simulink model "BMS_M0_pack_day4"  (R2026a)
settings: Solver=VariableStepAuto  AbsTol=1e-3  EnableMultiTasking=on
undefined symbols (not defined in the file or in its folder): bat, mcu
libraries: fl_lib x22, nesl_utility x18, batteryecm_lib x6, ee_lib x4, simulink x1
(part 2 of 2)

== matlab function BMS_M0_pack_day4/MATLAB Function ==
  data: cmd_preA output; tapsA input; cmd_mainA output; cmd_preB output; tapsB input; socA input; socB input; cmd_mainB output; cmd_load output; state_out output; fault_out output; Vbus input; iA input; iB input; dbg output; tempA input; tempB input
function [cmd_preA, cmd_mainA, cmd_preB, cmd_mainB, cmd_load, ...
          state_out, fault_out, dbg] = ...
         bms_reconfig_pass4(tapsA, tapsB, socA, socB, Vbus, iA, iB, ...
                            tempA, tempB)
%BMS_RECONFIG_PASS4  SOC/SOA-driven string-level reconfiguration controller.
%
%  ====================================================================
%  PROPRIETARY -- this file contains the novel contribution of this
%  project: dynamic string connect/disconnect/precharge for fault
%  isolation and SOC-driven wear levelling in a reconfigurable 3S2P pack.
%  Do not paste this logic into generic BMS code templates.
%  ====================================================================
%
%  MILESTONE 0 -- PASS 4 (final for M0).
%
%  REVISION HISTORY
%    Rev 1  SOA + topology logic.
%    Rev 2  Weld detection gated on precharge (Rev 1 tripped F_WELD_A on
%           startup because precharge current flows while the main pair is
%           deliberately open). SOC rejoin hysteresis actually applied --
%           Rev 1 rejoined at gap <= SPLIT_TH instead of < REJOIN_TH, so
%           the hysteresis band did nothing.
%    Rev 3  Warm-parallel guard reformulated. The 0.1 V rule is retained
%           for cold start, but under load the terminal difference between
%           strings is dominated by IR drop rather than stored-energy
%           mismatch, so it can never be satisfied. Bounded inrush is the
%           physically meaningful criterion. MEASURED Scenario 3: join at
%           dV = 0.149 V, inrush 1.5 A -> I_JOIN_MAX = 6 A gives 4x margin
%           while still blocking the 6.9 A cold-parallel case.
%    Rev 4  Overtemperature added (this file).
%
%  DESIGN RULES (from project brief, enforced in this order):
%    1. SOA checks run BEFORE any efficiency or balancing logic.
%    2. Break-before-make on every topology change.
%    3. Never parallel two strings unless the resulting inrush is bounded
%       (see Rev 3 note -- the original 0.1 V form is kept for cold start).
%    4. Minimum cooldown between topology changes (anti-oscillation).
%    5. Power-up / reset default is ALL SWITCHES OPEN.
%    6. Every switching action is validated by reading back current.
%
%  INPUTS
%    tapsA, tapsB  3x1  quantised tap voltages, referenced to pack negative
%    socA, socB    1x1  COULOMB-COUNTED estimates. Never true SOC.
%    Vbus          1x1  bus voltage (measured)
%    iA, iB        1x1  per-string current (measured, + = discharge)
%    tempA, tempB  3x1  per-cell temperature (deg C).
%                       INJECTED forcing function, not a thermal model --
%                       see M0 Day 1 scope decision. M0 makes NO claim
%                       about temperature reduction; that is bench-measured
%                       in M4.
%
%  OUTPUTS
%    cmd_preA/B    0/1  precharge bypass switch per string
%    cmd_mainA/B   0/1  main back-to-back pair per string
%    cmd_load      0/1  load disconnect switch
%    state_out          state code
%    fault_out          latched fault bitfield
%    dbg          10x1  diagnostics

%% ---- CONSTANTS ------------------------------------------------------
% KEEP IN SYNC WITH BMS_params.m -- a MATLAB Function block cannot read
% the base workspace.
DT              = 0.100;  % s   control loop period
V_UV_TRIP       = 2.50;   % V   [VERIFIED] SPEC pack design guideline, NCA
V_OV_TRIP       = 4.20;   % V   [VERIFIED] SPEC 3.3
I_OC_TRIP       = 12.0;   % A   [ASSUMPTION] per string, below the 15 A
                          %     cell rating with margin
T_OT_TRIP       = 60.0;   % C   [DESIGN] SPEC recommends re-discharge
                          %     release below 60 C. INTRO p.6 shows a 10 A
                          %     discharge reaching 60.9 C -- i.e. exactly
                          %     the single-string fault-mode operating
                          %     point, so this threshold is meaningful
                          %     rather than arbitrary.
T_OT_WARN       = 50.0;   % C   [ASSUMPTION] early-warning margin
DV_PARALLEL_MAX = 0.10;   % V   [ASSUMPTION] cold-start parallel limit
I_JOIN_MAX      = 6.0;    % A   [MEASURED-derived] Scenario 3 joined at
                          %     1.5 A; 6 A is 4x that and still blocks the
                          %     6.9 A unbalanced-warm-join case
R_STRING        = 0.100;  % ohm [CALCULATED] 3*20 mOhm cells + 2*20 mOhm
                          %     back-to-back MOSFET pair
T_COOLDOWN      = 0.50;   % s   [ASSUMPTION] min between topology changes
T_PRECHARGE_MAX = 0.50;   % s   [CALCULATED] 5*tau = 50 ms at R_pre = 10
                          %     ohm, C_bus = 1000 uF; 10x margin
VBUS_PRE_FRAC   = 0.95;   % fraction of string voltage = precharge done
SOC_SPLIT_TH    = 0.15;   % [DESIGN] gap at which we stop paralleling
SOC_REJOIN_TH   = 0.05;   % [DESIGN] hysteresis band for rejoining
DEBOUNCE_N      = 3;      % consecutive samples before a fault latches
VALIDATE_N      = 5;      % samples allowed for a switch to prove it moved
I_CONDUCT_MIN   = 0.20;   % A   above this counts as "current flowing"
STARTUP_N       = 10;     % ignore SOA for first 1 s while Simscape settles

%% ---- STATE CODES ----------------------------------------------------
S_INIT     = 0;   S_PRE_A    = 1;   S_PRE_B    = 2;
S_SINGLE_A = 3;   S_SINGLE_B = 4;   S_BOTH     = 5;
S_SHUTDOWN = 6;

%% ---- FAULT BITS -----------------------------------------------------
F_NONE   = 0;
F_UV_A   = 1;     F_UV_B   = 2;
F_OV_A   = 4;     F_OV_B   = 8;
F_OC_A   = 16;    F_OC_B   = 32;
F_PRE_A  = 64;    F_PRE_B  = 128;
F_WELD_A = 256;   F_WELD_B = 512;
F_OPEN_A = 1024;  F_OPEN_B = 2048;
F_OT_A   = 4096;  F_OT_B   = 8192;    % overtemperature

%% ---- PERSISTENT STATE ----------------------------------------------
persistent state fault
persistent uvA_c uvB_c ovA_c ovB_c ocA_c ocB_c otA_c otB_c
persistent t_state t_cool startup_c
persistent last_mainA last_mainB last_preA last_preB validate_c

if isempty(state)
    % POWER-UP DEFAULT: everything open. Mirrors the 100k base pull-downs
    % on the 2N2222A drivers -- on reset or brownout the hardware holds
    % the MOSFETs off, and the controller agrees.
    state = S_INIT;  fault = F_NONE;
    uvA_c = 0; uvB_c = 0; ovA_c = 0; ovB_c = 0;
    ocA_c = 0; ocB_c = 0; otA_c = 0; otB_c = 0;
    t_state = 0; t_cool = 0; startup_c = 0;
    last_mainA = 0; last_mainB = 0;
    last_preA  = 0; last_preB  = 0;
    validate_c = 0;
end

startup_c = startup_c + 1;
t_state   = t_state + DT;
if t_cool > 0, t_cool = t_cool - DT; end

%% ---- RECONSTRUCT PER-CELL VOLTAGES ---------------------------------
% The firmware performs this same subtraction: the dividers measure taps
% relative to pack negative, not individual cells. Measured reconstruction
% error 0.39 mV typical, ~7 mV worst case (2 LSB at 3.46 mV/LSB).
vA = [ tapsA(1); tapsA(2)-tapsA(1); tapsA(3)-tapsA(2) ];
vB = [ tapsB(1); tapsB(2)-tapsB(1); tapsB(3)-tapsB(2) ];

vStringA = tapsA(3);
vStringB = tapsB(3);

tMaxA = max(tempA);
tMaxB = max(tempB);

%% ---- STARTUP GRACE --------------------------------------------------
if startup_c < STARTUP_N
    cmd_preA = 0; cmd_mainA = 0;
    cmd_preB = 0; cmd_mainB = 0; cmd_load = 0;
    state_out = S_INIT; fault_out = F_NONE;
    dbg = [vA(1); vA(2); vA(3); vB(1); vB(2); vB(3); 0; 0; tMaxA; tMaxB];
    return
end

%% =====================================================================
%  LAYER 1 -- SOA CHECKS. These run first, always, and override
%  everything below.
%  =====================================================================
if any(vA < V_UV_TRIP),  uvA_c = uvA_c + 1; else, uvA_c = 0; end
if any(vB < V_UV_TRIP),  uvB_c = uvB_c + 1; else, uvB_c = 0; end
if any(vA > V_OV_TRIP),  ovA_c = ovA_c + 1; else, ovA_c = 0; end
if any(vB > V_OV_TRIP),  ovB_c = ovB_c + 1; else, ovB_c = 0; end
if abs(iA) > I_OC_TRIP,  ocA_c = ocA_c + 1; else, ocA_c = 0; end
if abs(iB) > I_OC_TRIP,  ocB_c = ocB_c + 1; else, ocB_c = 0; end
if tMaxA   > T_OT_TRIP,  otA_c = otA_c + 1; else, otA_c = 0; end
if tMaxB   > T_OT_TRIP,  otB_c = otB_c + 1; else, otB_c = 0; end

% Faults LATCH. An unloaded cell recovers voltage and would look healthy
% again; a cell removed from a heat source cools. Re-closing on either
% would oscillate the pack.
if uvA_c >= DEBOUNCE_N, fault = bitor(fault, F_UV_A); end
if uvB_c >= DEBOUNCE_N, fault = bitor(fault, F_UV_B); end
if ovA_c >= DEBOUNCE_N, fault = bitor(fault, F_OV_A); end
if ovB_c >= DEBOUNCE_N, fault = bitor(fault, F_OV_B); end
if ocA_c >= DEBOUNCE_N, fault = bitor(fault, F_OC_A); end
if ocB_c >= DEBOUNCE_N, fault = bitor(fault, F_OC_B); end
if otA_c >= DEBOUNCE_N, fault = bitor(fault, F_OT_A); end
if otB_c >= DEBOUNCE_N, fault = bitor(fault, F_OT_B); end

%% ---- STATE VALIDATION ----------------------------------------------
% A MOSFET welded closed is invisible to voltage sensing -- only current
% reveals it. Gate on the PREVIOUS cycle's precharge command: while a
% precharge switch is closed the main pair is deliberately open yet
% current legitimately flows through R_pre, which is otherwise
% indistinguishable from a weld.
in_precharge = (last_preA == 1) || (last_preB == 1);

if ~in_precharge && last_mainA == 0 && abs(iA) > I_CONDUCT_MIN
    fault = bitor(fault, F_WELD_A);
end
if ~in_precharge && last_mainB == 0 && abs(iB) > I_CONDUCT_MIN
    fault = bitor(fault, F_WELD_B);
end

% Commanded closed but no current -- only meaningful once the load is on
% and the state has settled.
if (state == S_BOTH || state == S_SINGLE_A) && last_mainA == 1 && ...
        abs(iA) < I_CONDUCT_MIN && t_state > 1.0
    validate_c = validate_c + 1;
    if validate_c >= VALIDATE_N, fault = bitor(fault, F_OPEN_A); end
elseif (state == S_BOTH || state == S_SINGLE_B) && last_mainB == 1 && ...
        abs(iB) < I_CONDUCT_MIN && t_state > 1.0
    validate_c = validate_c + 1;
    if validate_c >= VALIDATE_N, fault = bitor(fault, F_OPEN_B); end
else
    validate_c = 0;
end

faultA = bitand(fault, F_UV_A + F_OV_A + F_OC_A + F_OT_A + ...
                       F_PRE_A + F_WELD_A + F_OPEN_A) ~= 0;
faultB = bitand(fault, F_UV_B + F_OV_B + F_OC_B + F_OT_B + ...
                       F_PRE_B + F_WELD_B + F_OPEN_B) ~= 0;

%% =====================================================================
%  LAYER 2 -- BALANCING PREFERENCE (secondary; never overrides Layer 1)
%
%  A 2S string cannot be paralleled with a 3S string, so per-cell bypass
%  is unavailable. String-level selection is the only lever: run the
%  fuller string alone and let the emptier one rest.
%
%  MEASURED BEHAVIOUR (Scenario 3): from a 15% gap, single-string
%  operation closed the gap to 5% in 224 s, at which point the strings
%  rejoined. After rejoining the gap continued to zero WITHOUT controller
%  action -- paralleled strings self-balance through the bus. The value of
%  the split is therefore SAFE CONNECTION of mismatched strings, not extra
%  extracted energy. Do not claim the latter.
%  =====================================================================
soc_gap = socA - socB;
prefer_A_only = (soc_gap >  SOC_SPLIT_TH);
prefer_B_only = (soc_gap < -SOC_SPLIT_TH);
rejoin_ok     = (abs(soc_gap) < SOC_REJOIN_TH);

%% =====================================================================
%  LAYER 3 -- TRANSITION GUARDS
%  =====================================================================
% Cold start (load off, bus near 0 V): terminal dV is the right check.
% Warm parallel (load on): terminal dV is dominated by IR drop from the
% loaded string, not by stored-energy mismatch, so it can never fall below
% 0.1 V. Bound the resulting inrush instead -- that is the quantity the
% original rule was a proxy for.
dV_terminal = abs(vStringA - vStringB);
inrush_est  = dV_terminal / R_STRING;
dV_ok       = (dV_terminal < DV_PARALLEL_MAX) || (inrush_est < I_JOIN_MAX);

cool_ok   = (t_cool <= 0);
new_state = state;

switch state

    case S_INIT
        if     faultA && faultB, new_state = S_SHUTDOWN;
        elseif ~faultA,          new_state = S_PRE_A;
        elseif ~faultB,          new_state = S_PRE_B;
        else,                    new_state = S_SHUTDOWN;
        end

    case S_PRE_A
        % Bus charges through R_pre with the load disconnected. Only once
        % it has risen does the main pair close -- this is what keeps the
        % handover near 1 A instead of the measured 219 A cold-connect.
        if faultA
            new_state = S_SHUTDOWN;
        elseif Vbus >= VBUS_PRE_FRAC * vStringA
            new_state = S_SINGLE_A;
        elseif t_state > T_PRECHARGE_MAX
            fault = bitor(fault, F_PRE_A);
            new_state = S_SHUTDOWN;
        end

    case S_PRE_B
        if faultB
            new_state = S_SINGLE_A;
        elseif Vbus >= VBUS_PRE_FRAC * vStringB
            new_state = S_BOTH;
        elseif t_state > T_PRECHARGE_MAX
            fault = bitor(fault, F_PRE_B);
            new_state = S_SINGLE_A;
        end

    case S_SINGLE_A
        if     faultA && faultB,      new_state = S_SHUTDOWN;
        elseif faultA,                new_state = S_PRE_B;
        elseif ~faultB && cool_ok && dV_ok && rejoin_ok
                                      new_state = S_PRE_B;
        end

    case S_SINGLE_B
        if     faultA && faultB,      new_state = S_SHUTDOWN;
        elseif faultB,                new_state = S_PRE_A;
        elseif ~faultA && cool_ok && dV_ok && rejoin_ok
                                      new_state = S_PRE_A;
        end

    case S_BOTH
        if     faultA && faultB,         new_state = S_SHUTDOWN;
        elseif faultA,                   new_state = S_SINGLE_B;
        elseif faultB,                   new_state = S_SINGLE_A;
        elseif cool_ok && prefer_A_only, new_state = S_SINGLE_A;
        elseif cool_ok && prefer_B_only, new_state = S_SINGLE_B;
        end

    case S_SHUTDOWN
        % TERMINAL. Auto-recovery from an unknown fault is not defensible.

    otherwise
        new_state = S_SHUTDOWN;
end

if new_state ~= state
    state   = new_state;
    t_state = 0;
    t_cool  = T_COOLDOWN;
end

%% ---- OUTPUTS -------------------------------------------------------
% BREAK-BEFORE-MAKE is structural: no state asserts a precharge switch and
% its own main pair simultaneously.
switch state
    case S_INIT
        cmd_preA=0; cmd_mainA=0; cmd_preB=0; cmd_mainB=0; cmd_load=0;
    case S_PRE_A
        cmd_preA=1; cmd_mainA=0; cmd_preB=0; cmd_mainB=0; cmd_load=0;
    case S_SINGLE_A
        cmd_preA=0; cmd_mainA=1; cmd_preB=0; cmd_mainB=0; cmd_load=1;
    case S_PRE_B
        cmd_preA=0; cmd_mainA=1; cmd_preB=1; cmd_mainB=0; cmd_load=1;
    case S_SINGLE_B
        cmd_preA=0; cmd_mainA=0; cmd_preB=0; cmd_mainB=1; cmd_load=1;
    case S_BOTH
        cmd_preA=0; cmd_mainA=1; cmd_preB=0; cmd_mainB=1; cmd_load=1;
    case S_SHUTDOWN
        cmd_preA=0; cmd_mainA=0; cmd_preB=0; cmd_mainB=0; cmd_load=0;
    otherwise
        cmd_preA=0; cmd_mainA=0; cmd_preB=0; cmd_mainB=0; cmd_load=0;
end

last_mainA = cmd_mainA;  last_mainB = cmd_mainB;
last_preA  = cmd_preA;   last_preB  = cmd_preB;

state_out = state;
fault_out = fault;
dbg = [vA(1); vA(2); vA(3); vB(1); vB(2); vB(3); ...
       soc_gap; Vbus; tMaxA; tMaxB];

end

%% =====================================================================
%  FMEA -- PASS 4
%  =====================================================================
%
%  FAILURE                   DETECTION                   SAFE RESPONSE
%  --------------------------------------------------------------------
%  Cell undervoltage         cell < 2.50 V, 3 samples    Isolate string
%  Cell overvoltage          cell > 4.20 V, 3 samples    Isolate string
%  String overcurrent        |i| > 12 A, 3 samples       Isolate string
%  Cell overtemperature      T > 60 C, 3 samples         Isolate string
%
%  Internal cell short       Manifests as UV on that     Isolate string.
%  (the case a hard-          cell, and/or OT            Series topology
%   paralleled pack                                      means no loop
%   cannot address)                                      exists once the
%                                                        string switch is
%                                                        open. Measured
%                                                        leakage with the
%                                                        pair open:
%                                                        0.0004 mA.
%
%  MOSFET welded closed      commanded open but          Latch F_WELD;
%                            |i| > 0.2 A and not         cannot isolate,
%                            during precharge            so SHUTDOWN via
%                                                        load disconnect
%
%  MOSFET failed open        commanded closed but        Latch F_OPEN,
%                            |i| < 0.2 A, 5 samples      treat string as
%                                                        faulted
%
%  Single switch instead     N/A -- design-time.         MEASURED: a single
%  of a back-to-back pair    Body diode conducts.        switch leaked
%                                                        168,571 mA vs
%                                                        0.0004 mA for the
%                                                        pair. This is why
%                                                        the pair is
%                                                        mandatory.
%
%  Precharge resistor open   Vbus below 95% after        Latch F_PRE; do
%                            500 ms                      not close the main
%                                                        pair. Prevents the
%                                                        measured 218.8 A
%                                                        cold-connect.
%
%  Precharge switch welded   R_pre dissipates            NOT DETECTED.
%                            continuously                 [GAP -- needs a
%                                                        thermistor on
%                                                        R_pre or a
%                                                        separate i_pre
%                                                        measurement]
%
%  Both strings faulted      faultA && faultB            SHUTDOWN, load
%                                                        disconnected
%
%  Topology oscillation      T_COOLDOWN 500 ms +          Bounded to <= 2
%                            15%/5% SOC hysteresis        changes/second.
%                                                        MEASURED Scenario
%                                                        3: 6 transitions
%                                                        in 60 min.
%
%  Unsafe parallel join      inrush_est >= 6 A blocks    Transition blocked
%                            the transition               until the gap
%                                                        closes. MEASURED
%                                                        join: 1.5 A.
%
%  MCU reset mid-mission     persistents cleared          Re-enters S_INIT,
%                                                        all switches open;
%                                                        100k pull-downs
%                                                        hold the hardware
%                                                        off through reset
%
%  Coulomb counter drift     NOT DETECTED                 [KNOWN LIMITATION]
%                                                        MEASURED 5.06%
%                                                        after 10 min. SOC
%                                                        logic is secondary
%                                                        to SOA, so drift
%                                                        degrades balancing
%                                                        but never safety.
%
%  Capacity-fade lockout     NOT DETECTED                 [KNOWN GAP -- see
%  If one string accumulates                              below. Identified
%  more cycles its capacity                               during M0 review;
%  fades, so it reaches a                                 not yet mitigated]
%  given SOC faster. If the
%  capacities diverge far
%  enough the strings may
%  never satisfy rejoin_ok
%  simultaneously and the
%  pack locks permanently
%  into single-string
%  operation at half power.
%
%  KNOWN GAPS (M1 and beyond):
%    - Capacity-fade lockout, above. Mitigations to evaluate: track
%      cumulative Ah per string and favour the less-used string; or
%      compare capacity-normalised SOC rather than raw SOC in rejoin_ok.
%    - Precharge switch stuck-closed undetectable.
%    - Deliberate wear-levelling alternation not implemented. The SOC
%      split provides incidental alternation but is not driven by
%      cycle count.
%    - No thermal model. Temperature is an injected forcing function, so
%      M0 makes NO claim about temperature reduction. That is measured on
%      the bench in M4.
%    - Soft cell degradation is handled WORSE than a hard-paralleled pack:
%      isolating one weak cell costs the two healthy cells in its string.
%      State this trade-off explicitly rather than claiming general
%      superiority.
